simulink model "MCC"  (R2017b)
settings: Solver=ode15s  StartTime=0.0  StopTime=0.2  RelTol=1e-3
InitFcn:
  | MCC_constants
values from neighbouring files (symbols this model uses):
  b = 3.5077E-6    (= 3.5077e-06)    [MCC_constants.m]    (also in Td2.m = 0.0085; Tp3_data.m = 0.0085)
  Cr = 0    [MCC_constants.m]    (also in Td2.m; Tp3_data.m)
  J = 3.2284E-6    (= 3.2284e-06)    [MCC_constants.m]    (also in ProjetGiesData.m = 0.5; Td2.m = 0.28; Tp3_data.m = 0.2)
  K = 0.0274    [MCC_constants.m]    (also in Td2.m = 0.5093; Tp3_data.m = 0.9)
  L = 2.75E-6    (= 2.75e-06)    [MCC_constants.m]    (also in Td2.m = 0.0016; Tp3_data.m = 0.012161)
  R = 4    [MCC_constants.m]    (also in Td2.m = 0.13; Tp3_data.m = 0.895)
settings Model: Creator=Table2  LastModifiedBy=Table2

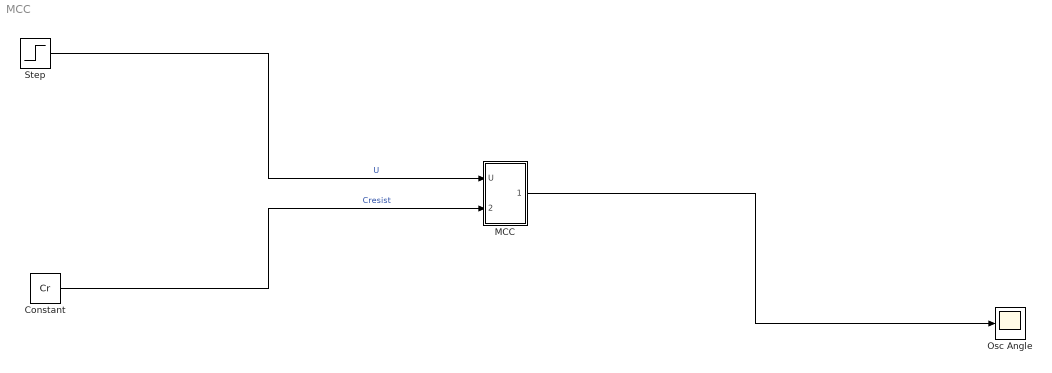
== system MCC ==
  Constant : Constant  Value=Cr
  MCC : Subsystem
  Osc Angle : Scope
  Step : Step  Time=0.01  After=12  SampleTime=0
  wires:
  Step/1 -> MCC/1(U)  "U"
  Constant/1 -> MCC/2(In2)  "Cresist"
  MCC/1(Out1) -> Osc Angle/1

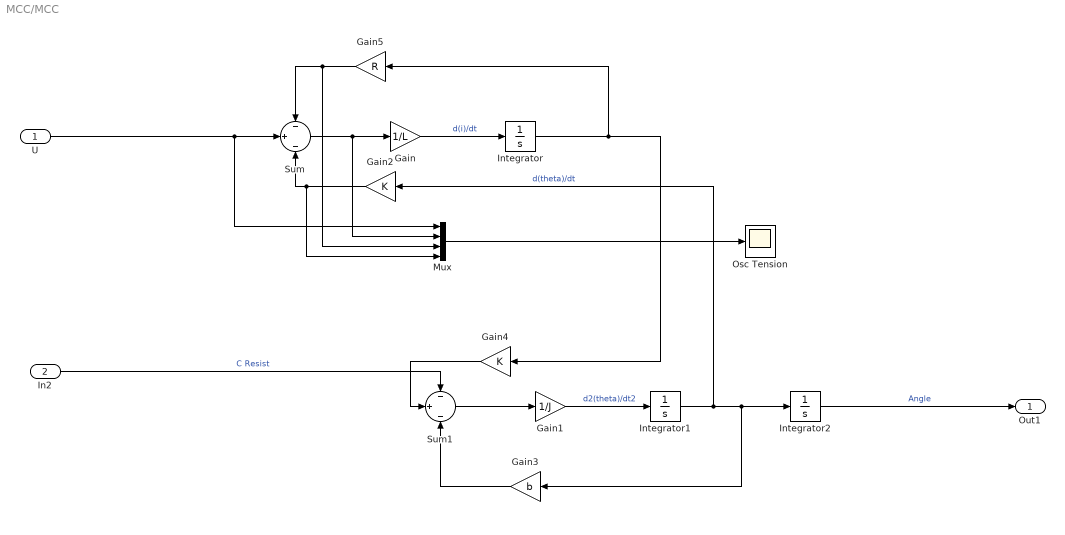
== system MCC/MCC ==
  U : Inport
  In2 : Inport  Port=2
  Gain : Gain  Gain=1/L
  Gain1 : Gain  Gain=1/J
  Gain2 : Gain  Gain=K
  Gain3 : Gain  Gain=b
  Gain4 : Gain  Gain=K
  Gain5 : Gain  Gain=R
  Integrator : Integrator
  Integrator1 : Integrator
  Integrator2 : Integrator
  Mux : Mux
  Osc Tension : Scope
  Sum : Sum  Inputs=-|+|-
  Sum1 : Sum  Inputs=-|+|-
  Out1 : Outport
  wires:
  Gain4/1 -> Sum1/2
  Gain3/1 -> Sum1/3
  Gain2/1 -> Mux/4, Sum/3
  Gain5/1 -> Mux/3, Sum/1
  In2/1 -> Sum1/1  "C Resist"
  Integrator/1 -> Gain5/1, Gain4/1
  Sum1/1 -> Gain1/1
  Gain1/1 -> Integrator1/1  "d2(theta)/dt2"
  Integrator1/1 -> Gain2/1, Gain3/1, Integrator2/1  "d(theta)/dt"
  Integrator2/1 -> Out1/1  "Angle"
  Mux/1 -> Osc Tension/1
  Sum/1 -> Mux/2, Gain/1
  U/1 -> Mux/1, Sum/2
  Gain/1 -> Integrator/1  "d(i)/dt"
